simulink subsystem "state_estimation"  (R2025b)
settings: Solver=VariableStepAuto  StartTime=0.0  StopTime=10.0  RelTol=1e-3
libraries: dspsrcs4 x1
settings Model: Creator=Aditya  LastModifiedBy=Aditya

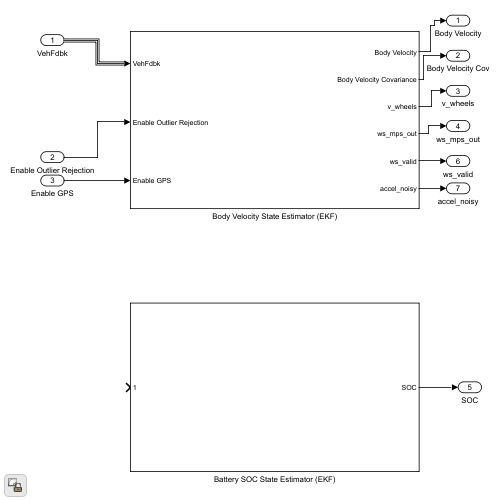
[thumbnail: Simulink's stored preview of the top-level diagram]
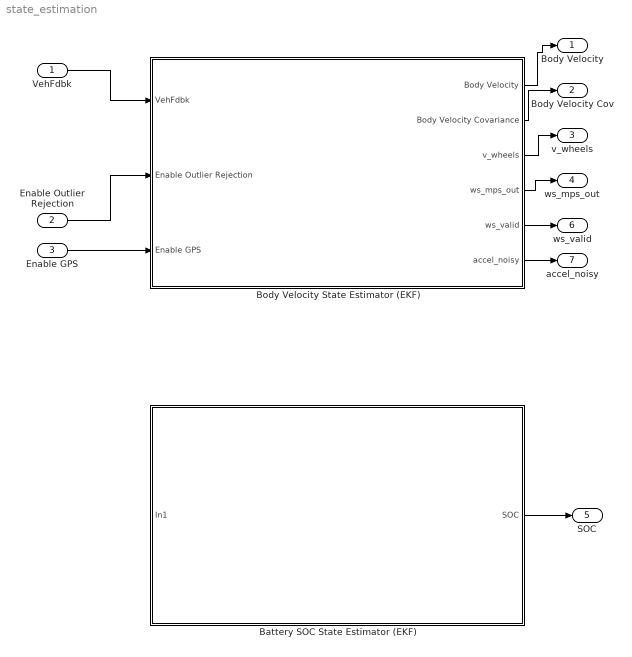
== system state_estimation ==
  VehFdbk : Inport
  Enable Outlier Rejection : Inport  Port=2
  Enable GPS : Inport  Port=3
  Battery SOC State Estimator (EKF) : Subsystem
  Body Velocity State Estimator (EKF) : Subsystem
  Body Velocity : Outport
  Body Velocity Cov : Outport  Port=2
  v_wheels : Outport  Port=3
  ws_mps_out : Outport  Port=4
  SOC : Outport  Port=5
  ws_valid : Outport  Port=6
  accel_noisy : Outport  Port=7
  wires:
  Body Velocity State Estimator (EKF)/1(Body Velocity) -> Body Velocity/1
  Battery SOC State Estimator (EKF)/1(SOC) -> SOC/1
  VehFdbk/1 -> Body Velocity State Estimator (EKF)/1(VehFdbk)
  Enable Outlier Rejection/1 -> Body Velocity State Estimator (EKF)/2(Enable Outlier Rejection)
  Enable GPS/1 -> Body Velocity State Estimator (EKF)/3(Enable GPS)
  Body Velocity State Estimator (EKF)/2(Body Velocity Covariance) -> Body Velocity Cov/1
  Body Velocity State Estimator (EKF)/3(v_wheels) -> v_wheels/1
  Body Velocity State Estimator (EKF)/4(ws_mps_out) -> ws_mps_out/1
  Body Velocity State Estimator (EKF)/5(ws_valid) -> ws_valid/1
  Body Velocity State Estimator (EKF)/6(accel_noisy) -> accel_noisy/1

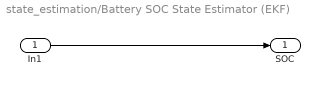
== system state_estimation/Battery SOC State Estimator (EKF) ==
  In1 : Inport
  SOC : Outport
  wires:
  In1/1 -> SOC/1

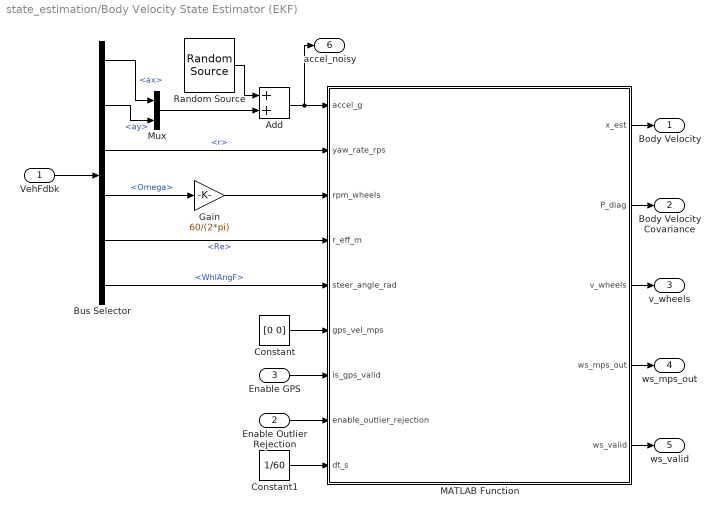
== system state_estimation/Body Velocity State Estimator (EKF) ==
  VehFdbk : Inport
  Enable Outlier Rejection : Inport  Port=2
  Enable GPS : Inport  Port=3
  Add : Sum
  Bus Selector : BusSelector  OutputSignals=BdyFrm.Cg.Acc.ax,BdyFrm.Cg.Acc.ay,BdyFrm.Cg.AngVel.r,Wheels.Omega,Wheels.Re,WhlAngF
  Constant : Constant  Value=[0 0]
  Constant1 : Constant  Value=1/60
  Gain : Gain  Gain=60/(2*pi)
  MATLAB Function : MATLAB Function  TreatAsAtomicUnit=on
  Mux : Mux  Inputs=2
  Random Source : dspsrcs4/Random Source  SrcType=Gaussian  MinVal=-0.5  MaxVal=0.5  MeanVal=0  VarVal=0.05/9.81  RepMode=Specify seed  rawSeed=1  IsInherit=on  SampTime=1  SampFrame=1  OutComplex=Real  DataType=double  SimulateUsing=Interpreted execution
  Body Velocity : Outport
  Body Velocity Covariance : Outport  Port=2
  v_wheels : Outport  Port=3
  ws_mps_out : Outport  Port=4
  ws_valid : Outport  Port=5
  accel_noisy : Outport  Port=6
  wires:
  Add/1 -> accel_noisy/1, MATLAB Function/1(accel_g)
  Random Source/1 -> Add/1
  Mux/1 -> Add/2
  MATLAB Function/4(ws_mps_out) -> ws_mps_out/1
  MATLAB Function/3(v_wheels) -> v_wheels/1
  Gain/1 -> MATLAB Function/3(rpm_wheels)
  MATLAB Function/2(P_diag) -> Body Velocity Covariance/1
  MATLAB Function/1(x_est) -> Body Velocity/1
  Constant1/1 -> MATLAB Function/9(dt_s)
  Constant/1 -> MATLAB Function/6(gps_vel_mps)
  Bus Selector/6 -> MATLAB Function/5(steer_angle_rad)  "<WhlAngF>"
  Bus Selector/5 -> MATLAB Function/4(r_eff_m)  "<Re>"
  Bus Selector/4 -> Gain/1  "<Omega>"
  Bus Selector/3 -> MATLAB Function/2(yaw_rate_rps)  "<r>"
  Bus Selector/2 -> Mux/2  "<ay>"
  Bus Selector/1 -> Mux/1  "<ax>"
  Enable GPS/1 -> MATLAB Function/7(is_gps_valid)
  Enable Outlier Rejection/1 -> MATLAB Function/8(enable_outlier_rejection)
  VehFdbk/1 -> Bus Selector/1
  MATLAB Function/5(ws_valid) -> ws_valid/1

== matlab function state_estimation/Body Velocity State Estimator (EKF)/MATLAB Function ==
  settings: updateMethod=DISCRETE
  data: accel_g input; x_est output; yaw_rate_rps input; rpm_wheels input; r_eff_m input; steer_angle_rad input; gps_vel_mps input; is_gps_valid input; enable_outlier_rejection input; dt_s input; P_diag output; v_wheels output; ws_mps_out output; ws_valid output
function [x_est, P_diag, v_wheels, ws_mps_out, ws_valid] = fcn( ...
        accel_g, yaw_rate_rps, rpm_wheels, r_eff_m, steer_angle_rad, ...
        gps_vel_mps, is_gps_valid, enable_outlier_rejection, dt_s)
%#codegen
% Body-frame velocity estimator (EKF)
%
% States:   x = [vx; vy]  (m/s, body frame)
%
% Inputs:
%   accel_g              [2x1]  Accelerometer (ax, ay) in g
%   yaw_rate_rps         [1x1]  Yaw rate (rad/s)
%   rpm_wheels           [4x1]  Wheel RPMs [FL; FR; RL; RR]
%   r_eff_m              [1x1]  Effective wheel radius (m)
%   steer_angle_rad      [2x1]  Front steer angles [delta_FL; delta_FR] (rad)
%   gps_vel_mps          [2x1]  GPS velocity [vx; vy] (m/s)
%   is_gps_valid         bool
%   enable_outlier_rejection  bool
%   dt_s                 [1x1]  Timestep (s)
%
% Outputs:
%   x_est       [2x1]  Estimated body velocity [vx; vy] (m/s)
%   P_diag      [2x1]  Diagonal of state covariance
%   v_wheels    [2x1]  Wheel-derived velocity measurement [vx; vy] (m/s)
%   ws_mps_out  [4x1]  Per-wheel linear speeds (m/s), for debug
%   ws_valid    bool   Whether wheel speed update was applied

    %% ---- Tuning & Configuration ----------------------------------------
    ENABLE_GPS_UPDATE = false;
    ENABLE_WS_UPDATE  = true;

    Q     = diag([0.01, 0.01]);   % Process noise covariance
    R_ws  = diag([100.0, 100.0]);   % Wheel speed measurement noise
    R_gps = diag([0.02, 0.02]);   % GPS measurement noise

    %% ---- Vehicle Parameters --------------------------------------------
    G_MPS2  = 9.81;
    TRACK_m = 1.100;
    Lf_m    = 0.807;
    Lr_m    = 1.554 - Lf_m;

    %% ---- Persistent State ----------------------------------------------
    persistent x P
    if isempty(x)
        x        = zeros(2,1);
        P        = eye(2);
    end

    %% ---- Unpack Inputs -------------------------------------------------
    ax = double(accel_g(1)) * G_MPS2;
    ay = double(accel_g(2)) * G_MPS2;
    wz = double(yaw_rate_rps);
    r  = double(r_eff_m);

    % Explicitly extract steer angles as scalars so codegen knows their size
    delta_fl = double(steer_angle_rad(1));
    delta_fr = double(steer_angle_rad(2));

    %% ---- 1. Predict ----------------------------------------------------
    % Body-frame kinematic model:
    %   vx_dot = ax + wz*vy
    %   vy_dot = ay - wz*vx
    x_dot = [ax + wz*x(2);
             ay - wz*x(1)];

    x = x + dt_s .* x_dot;
    x(1) = max(x(1), 0.0);

    % State transition Jacobian dF/dx
    F = [1,        dt_s*wz;
        -dt_s*wz,  1      ];

    P = F * P * F' + Q;

    %% ---- 2. Update: Wheel Speeds ---------------------------------------
    % Preallocate outputs with known fixed sizes for codegen
    v_wheels   = zeros(2,1);
    ws_mps_out = zeros(4,1);
    ws_valid   = false;

    if ENABLE_WS_UPDATE
        [z_ws, ws_valid, ws_mps_out] = wheelSpeedMeasurement( ...
            rpm_wheels, wz, delta_fl, delta_fr, r, ...
            TRACK_m, Lf_m, Lr_m, ...
            enable_outlier_rejection, x(1), ax);

        v_wheels  = z_ws;

        if ws_valid
            [x, P] = ekfUpdateH_I(x, P, z_ws, R_ws);
            x(1) = max(x(1), 0.0);
        end
    end

    %% ---- 3. Update: GPS -----------------------------------------------
    if ENABLE_GPS_UPDATE && is_gps_valid
        [x, P] = ekfUpdateH_I(x, P, gps_vel_mps, R_gps);
        x(1) = max(x(1), 0.0);
    end

    %% ---- Outputs -------------------------------------------------------
    x_est  = x;
    x_est(1) = max(x(1), 0.0);
    P_diag = [P(1,1); P(2,2)];
end


%% =========================================================================
function [x, P] = ekfUpdateH_I(x, P, z, R)
%#codegen
% EKF measurement update for H = I (measurement is directly the state)
    innov = z - x;      % Innovation          [2x1]
    S     = P + R;      % Innovation covariance (H=I => HPH' = P)
    K     = P / S;      % Kalman gain         [2x2]
    x     = x + K * innov;
    I = eye(2);
    P = (I - K)*P*(I - K)' + K*R*K';
end


%% =========================================================================
function [v_cg, valid, ws_mps] = wheelSpeedMeasurement( ...
        rpm, wz, delta_fl, delta_fr, r_eff, ...
        track, Lf, Lr, ...
        use_outlier, vx_ref, ax)
%#codegen
% Convert wheel RPMs to a body-frame CG velocity estimate.
% Wheel index convention: [FL; FR; RL; RR]

    %% ---- Constants -----------------------------------------------------
    V_MIN       = 0.5;    % (m/s) Denominator floor for slip ratio
    SLIP_THRESH = 0.117;   % Longitudinal slip threshold [0.1–0.3 typical]

    %% ---- Preallocate all fixed-size intermediates ----------------------
    % Required so Simulink codegen can infer output dimensions statically
    ws_mps = zeros(4,1);
    vx_w   = zeros(4,1);
    vy_w   = zeros(4,1);
    v_cg   = zeros(2,1);
    valid  = false;

    %% ---- Stopped vehicle shortcut -------------------------------------
    if all(rpm <= 0)
        valid = true;
        return;
    end

    %% ---- RPM -> wheel tangential speed (m/s) --------------------------
    k = r_eff * (2.0*pi / 60.0);
    ws_mps = rpm .* k;

    %% ---- Wheel contact-patch velocity -> body frame at CG -------------
    %
    % v_cg = R(delta) * v_wheel  +  wz x r_(wheel->CG)
    %
    ht = track * 0.5;

    c_fl = cos(delta_fl);   s_fl = sin(delta_fl);
    c_fr = cos(delta_fr);   s_fr = sin(delta_fr);

    % vx in body frame per wheel
    vx_w(1) = ws_mps(1)*c_fl + wz*ht;    % FL
    vx_w(2) = ws_mps(2)*c_fr - wz*ht;    % FR
    vx_w(3) = ws_mps(3)      + wz*ht;    % RL
    vx_w(4) = ws_mps(4)      - wz*ht;    % RR

    % vy in body frame per wheel
    vy_w(1) = ws_mps(1)*s_fl - wz*Lf;    % FL
    vy_w(2) = ws_mps(2)*s_fr - wz*Lf;    % FR
    vy_w(3) = wz*Lr;                      % RL
    vy_w(4) = wz*Lr;                      % RR

    %% ---- Outlier Rejection + Averaging --------------------------------
    % Use explicit loop (no logical indexing) so codegen sees fixed sizes
    den    = max(V_MIN, abs(vx_ref));
    sum_vx = 0.0;
    sum_vy = 0.0;
    count  = 0;

    % Longitudinal wheel speed projected to body x-axis (for slip check)
    vwx_long = zeros(4,1);
    vwx_long(1) = ws_mps(1) * c_fl;
    vwx_long(2) = ws_mps(2) * c_fr;
    vwx_long(3) = ws_mps(3);
    vwx_long(4) = ws_mps(4);

    for i = 1:4
        include = true;

        if use_outlier
            % Reject on excessive longitudinal slip
            slip = (vwx_long(i) - vx_ref) / den;
            if slip > SLIP_THRESH || slip < -SLIP_THRESH
                include = false;
            end
        end

        if include
            sum_vx = sum_vx + vx_w(i);
            sum_vy = sum_vy + vy_w(i);
            count  = count + 1;
        end
    end

    %% ---- Output -------------------------------------------------------
    if count > 0
        v_cg(1) = sum_vx / count;
        v_cg(2) = sum_vy / count;
        valid   = true;
    end
end
